simulink model "sm_DynamicCompression"  (R2019b)
settings: Solver=FixedStepDiscrete  StartTime=0.0  StopTime=stop_time  RelTol=1e-3
InitFcn:
  | sm_callback_init
StopFcn:
  | sm_callback_stop
values from neighbouring files (symbols this model uses):
  a = 100*(r^2)    [InitializeCompressionSettings.m]    (also in sm_check_control_signals.m = registers(i).(supplied_fields{j}); sm_check_control_signals_LOCAL_1434.m = registers(i).(supplied_fields{j}))
  B_k_0_init = zeros(1,FIR_0_Uprate)    [sm_callback_init.m]
  B_k_1_init = zeros(1,FIR_0_Uprate)    [sm_callback_init.m]
  B_k_2_init = zeros(1,FIR_0_Uprate)    [sm_callback_init.m]
  B_k_3_init = zeros(1,FIR_0_Uprate)    [sm_callback_init.m]
  B_k_4_init = zeros(1,FIR_0_Uprate)    [sm_callback_init.m]
  B_k_5_init = zeros(1,FIR_0_Uprate)    [sm_callback_init.m]
  calib_bpfs = bpfs    [sm_compression_init.m]
  delayFix = maxDelay-delays    [Initialize_Delay_Values.m]
  F_bits = 28    [TestingLibraryScripts.m]    (also in sm_compression_init.m)
  FIR_0_Size = (ceil(log2(length(calib_bpfs(2:calib_bpfs(1,1)+1 ,1)'))))    [sm_callback_init.m]
  FIR_0_Uprate = 2^FIR_0_Size    [sm_callback_init.m]
  M_bits = 1    [TestingLibraryScripts.m]    (also in sm_compression_init.m = 5)
  M_Bits = M_bits    (= 5)    [sm_compression_init.m]
  mp = sm_init_avalon_signals(mp)    [sm_callback_init.m]
  r_att = nthroot(0.1, s_att)    [sm_compression_init.m]
  r_rel = nthroot(0.1, s_rel)    [sm_compression_init.m]
  recombGain = ones(1,NChans)    [sm_compression_init.m]
  TABLE_SEL_BYPASS_ENABLE = 0    [sm_callback_init.m]
  Ts = mp.Ts    [sm_compression_init.m]
  Ts_system = mp.Ts_system    [sm_compression_init.m]
  W_bits = 32    [TestingLibraryScripts.m]    (also in sm_compression_init.m)
  X_high = 1    [sm_compression_init.m]
undefined symbols (not defined in the file or in its folder): b, c, Gain_Table, ig_eq
libraries: hdlsllib x272, simulink x127, dsphdlfiltering x2
(part 3 of 8)

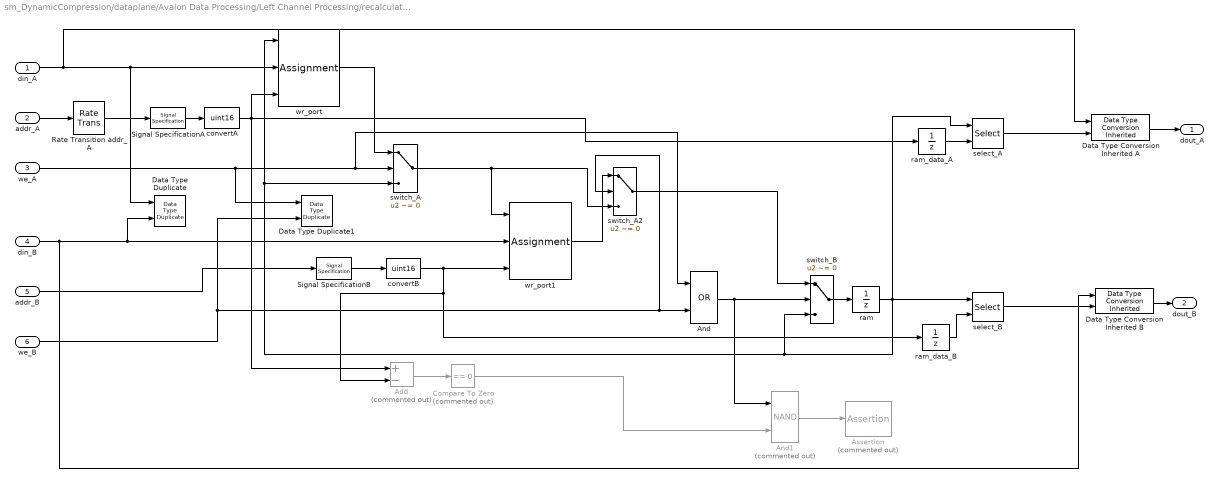
== system sm_DynamicCompression/dataplane/Avalon Data Processing/Left Channel Processing/recalculate/Nchan_FbankAGC_AID/Static_pFIR/Input_Data_Circular_Buffer_old ==
  din_A : Inport
  addr_A : Inport  Port=2
  we_A : Inport  Port=3  OutDataTypeStr=boolean
  din_B : Inport  Port=4
  addr_B : Inport  Port=5
  we_B : Inport  Port=6  OutDataTypeStr=boolean
  Add : Sum  Commented=on  Inputs=+-
  And : Logic  Operator=OR  AllPortsSameDT=off  OutDataTypeStr=boolean
  And1 : Logic  Commented=on  Operator=NAND  AllPortsSameDT=off  OutDataTypeStr=boolean
  Assertion : Assertion  Commented=on  StopWhenAssertionFail=off
  Compare To Zero : simulink/Logic and Bit Operations/Compare To Zero  Commented=on  relop===  OutDataTypeStr=boolean
  Data Type Conversion Inherited A : simulink/Signal Attributes/Data Type Conversion Inherited  ConvertRealWorld=Real World Value  DoSatur=off
      settings: SourceProductName=Simulink  SourceProductBaseCode=SL
  Data Type Conversion Inherited B : simulink/Signal Attributes/Data Type Conversion Inherited  ConvertRealWorld=Real World Value  DoSatur=off
      settings: SourceProductName=Simulink  SourceProductBaseCode=SL
  Data Type Duplicate : DataTypeDuplicate
  Data Type Duplicate1 : DataTypeDuplicate
  Rate Transition addr_A : RateTransition
  Signal SpecificationA : SignalSpecification  OutDataTypeStr=fixdt(0,ram_size,0)  Dimensions=1
  Signal SpecificationB : SignalSpecification  OutDataTypeStr=fixdt(0,ram_size,0)  Dimensions=1
  convertA : DataTypeConversion  OutDataTypeStr=uint16
  convertB : DataTypeConversion  OutDataTypeStr=uint16
  ram : UnitDelay  SampleTime=-1  HasFrameUpgradeWarning=on
  ram_data_A : UnitDelay  SampleTime=-1  HasFrameUpgradeWarning=on
  ram_data_B : UnitDelay  SampleTime=-1  HasFrameUpgradeWarning=on
  select_A : Selector  IndexMode=Zero-based  InputPortWidth=2^ram_size  IndexOptions=Index vector (port)  Indices=[1 3]  OutputSizes=1
  select_B : Selector  IndexMode=Zero-based  InputPortWidth=2^ram_size  IndexOptions=Index vector (port)  Indices=[1 3]  OutputSizes=1
  switch_A : Switch  Criteria=u2 ~= 0
  switch_A2 : Switch  Criteria=u2 ~= 0
  switch_B : Switch  Criteria=u2 ~= 0
  wr_port : Assignment  IndexMode=Zero-based  IndexOptions=Index vector (port)  Indices=1  OutputSizes=[1 1]
  wr_port1 : Assignment  IndexMode=Zero-based  IndexOptions=Index vector (port)  Indices=1  OutputSizes=[1 1]
  dout_A : Outport  VectorParamsAs1DForOutWhenUnconnected=off
  dout_B : Outport  Port=2  VectorParamsAs1DForOutWhenUnconnected=off
  wires:
  Data Type Conversion Inherited A/1 -> dout_A/1
  select_A/1 -> Data Type Conversion Inherited A/2
  Data Type Conversion Inherited B/1 -> dout_B/1
  select_B/1 -> Data Type Conversion Inherited B/2
  Rate Transition addr_A/1 -> Signal SpecificationA/1
  addr_A/1 -> Rate Transition addr_A/1
  din_B/1 -> Data Type Duplicate/2, wr_port1/2, Data Type Conversion Inherited B/1
  convertB/1 -> wr_port1/3, Add/2, ram_data_B/1
  din_A/1 -> wr_port/2, Data Type Duplicate/1, Data Type Conversion Inherited A/1
  ram_data_A/1 -> select_A/2
  we_A/1 -> switch_A/2, And/1, Data Type Duplicate1/1
  ram_data_B/1 -> select_B/2
  addr_B/1 -> Signal SpecificationB/1
  switch_A/1 -> switch_A2/3, wr_port1/1
  we_B/1 -> Data Type Duplicate1/2, And/2, switch_A2/2
  Compare To Zero/1 -> And1/2
  Add/1 -> Compare To Zero/1
  wr_port1/1 -> switch_A2/1
  And/1 -> switch_B/2, And1/1
  wr_port/1 -> switch_A/1
  ram/1 -> select_A/1, wr_port/1, switch_A/3, switch_B/3, select_B/1
  convertA/1 -> Add/1, wr_port/3, ram_data_A/1
  switch_B/1 -> ram/1
  Signal SpecificationB/1 -> convertB/1
  Signal SpecificationA/1 -> convertA/1
  And1/1 -> Assertion/1
  switch_A2/1 -> switch_B/1

== system sm_DynamicCompression/dataplane/Avalon Data Processing/Left Channel Processing/recalculate/Nchan_FbankAGC_AID/Static_pFIR/Multiply_And_Sum ==
  note: Try to use this at some point?
  note: End_of_sample_calc triggers this subsystem to give the FIR output for this sample.
      | Also, it resets the sum memory back to 0.
  x[n-i] : Inport
  End_of_sample_calc : Inport  Port=2
  b_i : Inport  Port=3
  Bitwise Operator : simulink/Logic and Bit Operations/Bitwise Operator  logicop=NOT  UseBitMask=off  BitMask=bin2dec('11011001')  BitMaskRealWorld=Stored Integer
  Constant : Constant  Value=0  OutDataTypeStr=fixdt(1, W_bits, F_bits)  SampleTime=Ts/FIR_0_Uprate
  Multiply-Add : hdlsllib/HDL Operations/Multiply-Add  Function=c+(a.*b)  datatype=Inherit: Same as first input  DoSatur=off  FMA=off
      settings: SourceProductName=Simulink  SourceProductBaseCode=SL
  Reset_Switch : Switch  Criteria=u2 ~= 0  ZeroCross=off
  Sum_memory : UnitDelay  SampleTime=-1  HasFrameUpgradeWarning=on
  Filtered_Output : Outport  VectorParamsAs1DForOutWhenUnconnected=off
  Output_Valid : Outport  Port=2  VectorParamsAs1DForOutWhenUnconnected=off
  wires:
  x[n-i]/1 -> Multiply-Add/1
  End_of_sample_calc/1 -> Output_Valid/1, Bitwise Operator/1
  b_i/1 -> Multiply-Add/2
  Sum_memory/1 -> Multiply-Add/3, Filtered_Output/1
  Multiply-Add/1 -> Reset_Switch/1
  Reset_Switch/1 -> Sum_memory/1
  Constant/1 -> Reset_Switch/3
  Bitwise Operator/1 -> Reset_Switch/2

== system sm_DynamicCompression/dataplane/Avalon Data Processing/Left Channel Processing/recalculate/Nchan_FbankAGC_AID/Static_pFIR1/Addr_Gen  ==
  note: Realign Delay here?
  Add : Sum  OutDataTypeStr=Inherit: Same as first input
  Compare To Zero : simulink/Logic and Bit Operations/Compare To Zero  relop===  OutDataTypeStr=boolean  ZeroCross=off
  Constant : Constant  OutDataTypeStr=fixdt(0, FIR_0_Size,0)  SampleTime=-1
  Counter 0 to |b_k|-1 : simulink/Sources/Counter Free-Running  NumBits=FIR_0_Size  tsamp=Ts/FIR_0_Uprate
  Input_Addr_Counter : simulink/Sources/Counter Free-Running  NumBits=FIR_0_Size  tsamp=Ts
  Rate Transition : RateTransition  OutPortSampleTime=Ts/FIR_0_Uprate
  Realignment_delay : Constant  Value=delayFix(2)  OutDataTypeStr=fixdt(0, FIR_0_Size,0)  SampleTime=-1
  Subtract : Sum  Inputs=+--  OutDataTypeStr=Inherit: Same as first input
  Input_Addr : Outport  VectorParamsAs1DForOutWhenUnconnected=off
  Data_History_Rd_addr : Outport  Port=2  VectorParamsAs1DForOutWhenUnconnected=off
  End_of_sample_calc : Outport  Port=3  VectorParamsAs1DForOutWhenUnconnected=off
  b_k_addr : Outport  Port=4  VectorParamsAs1DForOutWhenUnconnected=off
  wires:
  Rate Transition/1 -> Add/1, Subtract/1
  Compare To Zero/1 -> End_of_sample_calc/1
  Realignment_delay/1 -> Subtract/3
  Constant/1 -> Add/2
  Add/1 -> Input_Addr/1
  Input_Addr_Counter/1 -> Rate Transition/1
  Subtract/1 -> Data_History_Rd_addr/1
  Counter 0 to |b_k|-1/1 -> b_k_addr/1, Compare To Zero/1, Subtract/2

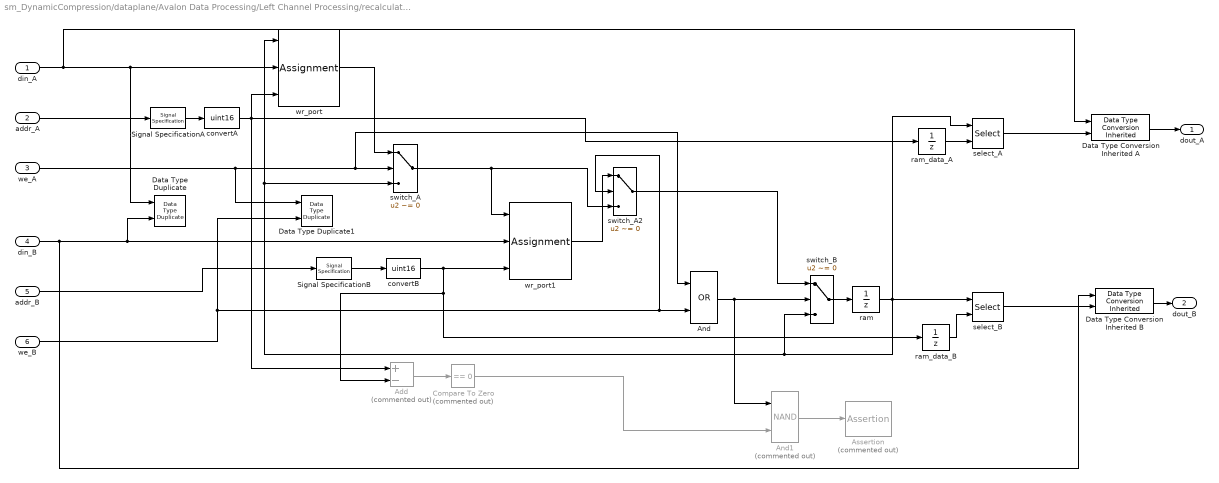
== system sm_DynamicCompression/dataplane/Avalon Data Processing/Left Channel Processing/recalculate/Nchan_FbankAGC_AID/Static_pFIR1/B_k_Memory_Block ==
  din_A : Inport
  addr_A : Inport  Port=2
  we_A : Inport  Port=3  OutDataTypeStr=boolean
  din_B : Inport  Port=4
  addr_B : Inport  Port=5
  we_B : Inport  Port=6  OutDataTypeStr=boolean
  Add : Sum  Commented=on  Inputs=+-
  And : Logic  Operator=OR  AllPortsSameDT=off  OutDataTypeStr=boolean
  And1 : Logic  Commented=on  Operator=NAND  AllPortsSameDT=off  OutDataTypeStr=boolean
  Assertion : Assertion  Commented=on  StopWhenAssertionFail=off
  Compare To Zero : simulink/Logic and Bit Operations/Compare To Zero  Commented=on  relop===  OutDataTypeStr=boolean
  Data Type Conversion Inherited A : simulink/Signal Attributes/Data Type Conversion Inherited  ConvertRealWorld=Real World Value  DoSatur=off
      settings: SourceProductName=Simulink  SourceProductBaseCode=SL
  Data Type Conversion Inherited B : simulink/Signal Attributes/Data Type Conversion Inherited  ConvertRealWorld=Real World Value  DoSatur=off
      settings: SourceProductName=Simulink  SourceProductBaseCode=SL
  Data Type Duplicate : DataTypeDuplicate
  Data Type Duplicate1 : DataTypeDuplicate
  Signal SpecificationA : SignalSpecification  OutDataTypeStr=fixdt(0,ram_size,0)  Dimensions=1
  Signal SpecificationB : SignalSpecification  OutDataTypeStr=fixdt(0,ram_size,0)  Dimensions=1
  convertA : DataTypeConversion  OutDataTypeStr=uint16
  convertB : DataTypeConversion  OutDataTypeStr=uint16
  ram : UnitDelay  InitialCondition=B_k_1_init  SampleTime=-1  HasFrameUpgradeWarning=on
  ram_data_A : UnitDelay  SampleTime=-1  HasFrameUpgradeWarning=on
  ram_data_B : UnitDelay  SampleTime=-1  HasFrameUpgradeWarning=on
  select_A : Selector  IndexMode=Zero-based  InputPortWidth=2^ram_size  IndexOptions=Index vector (port)  Indices=[1 3]  OutputSizes=1
  select_B : Selector  IndexMode=Zero-based  InputPortWidth=2^ram_size  IndexOptions=Index vector (port)  Indices=[1 3]  OutputSizes=1
  switch_A : Switch  Criteria=u2 ~= 0
  switch_A2 : Switch  Criteria=u2 ~= 0
  switch_B : Switch  Criteria=u2 ~= 0
  wr_port : Assignment  IndexMode=Zero-based  IndexOptions=Index vector (port)  Indices=1  OutputSizes=[1 1]
  wr_port1 : Assignment  IndexMode=Zero-based  IndexOptions=Index vector (port)  Indices=1  OutputSizes=[1 1]
  dout_A : Outport  VectorParamsAs1DForOutWhenUnconnected=off
  dout_B : Outport  Port=2  VectorParamsAs1DForOutWhenUnconnected=off
  wires:
  Data Type Conversion Inherited A/1 -> dout_A/1
  select_A/1 -> Data Type Conversion Inherited A/2
  Data Type Conversion Inherited B/1 -> dout_B/1
  select_B/1 -> Data Type Conversion Inherited B/2
  addr_A/1 -> Signal SpecificationA/1
  din_B/1 -> Data Type Conversion Inherited B/1, Data Type Duplicate/2, wr_port1/2
  convertB/1 -> wr_port1/3, Add/2, ram_data_B/1
  din_A/1 -> Data Type Conversion Inherited A/1, wr_port/2, Data Type Duplicate/1
  ram_data_A/1 -> select_A/2
  we_A/1 -> switch_A/2, And/1, Data Type Duplicate1/1
  ram_data_B/1 -> select_B/2
  addr_B/1 -> Signal SpecificationB/1
  switch_A/1 -> switch_A2/3, wr_port1/1
  we_B/1 -> Data Type Duplicate1/2, And/2, switch_A2/2
  Compare To Zero/1 -> And1/2
  Add/1 -> Compare To Zero/1
  wr_port1/1 -> switch_A2/1
  And/1 -> switch_B/2, And1/1
  wr_port/1 -> switch_A/1
  ram/1 -> select_A/1, wr_port/1, switch_A/3, switch_B/3, select_B/1
  convertA/1 -> Add/1, wr_port/3, ram_data_A/1
  switch_B/1 -> ram/1
  Signal SpecificationB/1 -> convertB/1
  Signal SpecificationA/1 -> convertA/1
  And1/1 -> Assertion/1
  switch_A2/1 -> switch_B/1

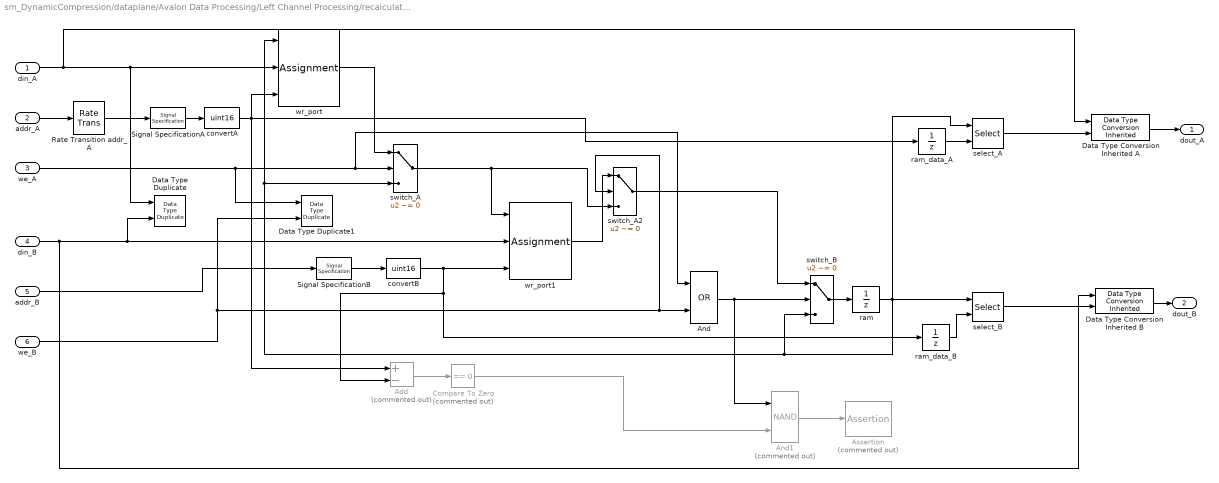
== system sm_DynamicCompression/dataplane/Avalon Data Processing/Left Channel Processing/recalculate/Nchan_FbankAGC_AID/Static_pFIR1/Input_Data_Circular_Buffer_old ==
  din_A : Inport
  addr_A : Inport  Port=2
  we_A : Inport  Port=3  OutDataTypeStr=boolean
  din_B : Inport  Port=4
  addr_B : Inport  Port=5
  we_B : Inport  Port=6  OutDataTypeStr=boolean
  Add : Sum  Commented=on  Inputs=+-
  And : Logic  Operator=OR  AllPortsSameDT=off  OutDataTypeStr=boolean
  And1 : Logic  Commented=on  Operator=NAND  AllPortsSameDT=off  OutDataTypeStr=boolean
  Assertion : Assertion  Commented=on  StopWhenAssertionFail=off
  Compare To Zero : simulink/Logic and Bit Operations/Compare To Zero  Commented=on  relop===  OutDataTypeStr=boolean
  Data Type Conversion Inherited A : simulink/Signal Attributes/Data Type Conversion Inherited  ConvertRealWorld=Real World Value  DoSatur=off
      settings: SourceProductName=Simulink  SourceProductBaseCode=SL
  Data Type Conversion Inherited B : simulink/Signal Attributes/Data Type Conversion Inherited  ConvertRealWorld=Real World Value  DoSatur=off
      settings: SourceProductName=Simulink  SourceProductBaseCode=SL
  Data Type Duplicate : DataTypeDuplicate
  Data Type Duplicate1 : DataTypeDuplicate
  Rate Transition addr_A : RateTransition
  Signal SpecificationA : SignalSpecification  OutDataTypeStr=fixdt(0,ram_size,0)  Dimensions=1
  Signal SpecificationB : SignalSpecification  OutDataTypeStr=fixdt(0,ram_size,0)  Dimensions=1
  convertA : DataTypeConversion  OutDataTypeStr=uint16
  convertB : DataTypeConversion  OutDataTypeStr=uint16
  ram : UnitDelay  SampleTime=-1  HasFrameUpgradeWarning=on
  ram_data_A : UnitDelay  SampleTime=-1  HasFrameUpgradeWarning=on
  ram_data_B : UnitDelay  SampleTime=-1  HasFrameUpgradeWarning=on
  select_A : Selector  IndexMode=Zero-based  InputPortWidth=2^ram_size  IndexOptions=Index vector (port)  Indices=[1 3]  OutputSizes=1
  select_B : Selector  IndexMode=Zero-based  InputPortWidth=2^ram_size  IndexOptions=Index vector (port)  Indices=[1 3]  OutputSizes=1
  switch_A : Switch  Criteria=u2 ~= 0
  switch_A2 : Switch  Criteria=u2 ~= 0
  switch_B : Switch  Criteria=u2 ~= 0
  wr_port : Assignment  IndexMode=Zero-based  IndexOptions=Index vector (port)  Indices=1  OutputSizes=[1 1]
  wr_port1 : Assignment  IndexMode=Zero-based  IndexOptions=Index vector (port)  Indices=1  OutputSizes=[1 1]
  dout_A : Outport  VectorParamsAs1DForOutWhenUnconnected=off
  dout_B : Outport  Port=2  VectorParamsAs1DForOutWhenUnconnected=off
  wires:
  switch_A2/1 -> switch_B/1
  And1/1 -> Assertion/1
  Signal SpecificationA/1 -> convertA/1
  Signal SpecificationB/1 -> convertB/1
  switch_B/1 -> ram/1
  convertA/1 -> ram_data_A/1, wr_port/3, Add/1
  ram/1 -> select_B/1, switch_B/3, switch_A/3, wr_port/1, select_A/1
  wr_port/1 -> switch_A/1
  And/1 -> And1/1, switch_B/2
  wr_port1/1 -> switch_A2/1
  Add/1 -> Compare To Zero/1
  Compare To Zero/1 -> And1/2
  we_B/1 -> switch_A2/2, And/2, Data Type Duplicate1/2
  switch_A/1 -> wr_port1/1, switch_A2/3
  addr_B/1 -> Signal SpecificationB/1
  ram_data_B/1 -> select_B/2
  we_A/1 -> Data Type Duplicate1/1, And/1, switch_A/2
  ram_data_A/1 -> select_A/2
  din_A/1 -> Data Type Conversion Inherited A/1, Data Type Duplicate/1, wr_port/2
  convertB/1 -> ram_data_B/1, Add/2, wr_port1/3
  din_B/1 -> Data Type Conversion Inherited B/1, wr_port1/2, Data Type Duplicate/2
  addr_A/1 -> Rate Transition addr_A/1
  Rate Transition addr_A/1 -> Signal SpecificationA/1
  select_B/1 -> Data Type Conversion Inherited B/2
  Data Type Conversion Inherited B/1 -> dout_B/1
  select_A/1 -> Data Type Conversion Inherited A/2
  Data Type Conversion Inherited A/1 -> dout_A/1

== system sm_DynamicCompression/dataplane/Avalon Data Processing/Left Channel Processing/recalculate/Nchan_FbankAGC_AID/Static_pFIR1/Multiply_And_Sum ==
  note: End_of_sample_calc triggers this subsystem to give the FIR output for this sample.
      | Also, it resets the sum memory back to 0.
  note: Try to use this at some point?
  x[n-i] : Inport
  End_of_sample_calc : Inport  Port=2
  b_i : Inport  Port=3
  Bitwise Operator : simulink/Logic and Bit Operations/Bitwise Operator  logicop=NOT  UseBitMask=off  BitMask=bin2dec('11011001')  BitMaskRealWorld=Stored Integer
  Constant : Constant  Value=0  OutDataTypeStr=fixdt(1, W_bits, F_bits)  SampleTime=Ts/FIR_0_Uprate
  Multiply-Add : hdlsllib/HDL Operations/Multiply-Add  Function=c+(a.*b)  datatype=Inherit: Same as first input  DoSatur=off  FMA=off
      settings: SourceProductName=Simulink  SourceProductBaseCode=SL
  Reset_Switch : Switch  Criteria=u2 ~= 0  ZeroCross=off
  Sum_memory : UnitDelay  SampleTime=-1  HasFrameUpgradeWarning=on
  Filtered_Output : Outport  VectorParamsAs1DForOutWhenUnconnected=off
  Output_Valid : Outport  Port=2  VectorParamsAs1DForOutWhenUnconnected=off
  wires:
  Bitwise Operator/1 -> Reset_Switch/2
  Constant/1 -> Reset_Switch/3
  Reset_Switch/1 -> Sum_memory/1
  Multiply-Add/1 -> Reset_Switch/1
  Sum_memory/1 -> Filtered_Output/1, Multiply-Add/3
  b_i/1 -> Multiply-Add/2
  End_of_sample_calc/1 -> Bitwise Operator/1, Output_Valid/1
  x[n-i]/1 -> Multiply-Add/1

== system sm_DynamicCompression/dataplane/Avalon Data Processing/Left Channel Processing/recalculate/Nchan_FbankAGC_AID/Static_pFIR2/Addr_Gen  ==
  note: Realign Delay here?
  Add : Sum  OutDataTypeStr=Inherit: Same as first input
  Compare To Zero : simulink/Logic and Bit Operations/Compare To Zero  relop===  OutDataTypeStr=boolean  ZeroCross=off
  Constant : Constant  OutDataTypeStr=fixdt(0, FIR_0_Size,0)  SampleTime=-1
  Counter 0 to |b_k|-1 : simulink/Sources/Counter Free-Running  NumBits=FIR_0_Size  tsamp=Ts/FIR_0_Uprate
  Input_Addr_Counter : simulink/Sources/Counter Free-Running  NumBits=FIR_0_Size  tsamp=Ts
  Rate Transition : RateTransition  OutPortSampleTime=Ts/FIR_0_Uprate
  Realignment_delay : Constant  Value=delayFix(3)  OutDataTypeStr=fixdt(0, FIR_0_Size,0)  SampleTime=-1
  Subtract : Sum  Inputs=+--  OutDataTypeStr=Inherit: Same as first input
  Input_Addr : Outport  VectorParamsAs1DForOutWhenUnconnected=off
  Data_History_Rd_addr : Outport  Port=2  VectorParamsAs1DForOutWhenUnconnected=off
  End_of_sample_calc : Outport  Port=3  VectorParamsAs1DForOutWhenUnconnected=off
  b_k_addr : Outport  Port=4  VectorParamsAs1DForOutWhenUnconnected=off
  wires:
  Counter 0 to |b_k|-1/1 -> Subtract/2, Compare To Zero/1, b_k_addr/1
  Subtract/1 -> Data_History_Rd_addr/1
  Input_Addr_Counter/1 -> Rate Transition/1
  Add/1 -> Input_Addr/1
  Constant/1 -> Add/2
  Realignment_delay/1 -> Subtract/3
  Compare To Zero/1 -> End_of_sample_calc/1
  Rate Transition/1 -> Subtract/1, Add/1

== system sm_DynamicCompression/dataplane/Avalon Data Processing/Left Channel Processing/recalculate/Nchan_FbankAGC_AID/Static_pFIR2/B_k_Memory_Block ==
  din_A : Inport
  addr_A : Inport  Port=2
  we_A : Inport  Port=3  OutDataTypeStr=boolean
  din_B : Inport  Port=4
  addr_B : Inport  Port=5
  we_B : Inport  Port=6  OutDataTypeStr=boolean
  Add : Sum  Commented=on  Inputs=+-
  And : Logic  Operator=OR  AllPortsSameDT=off  OutDataTypeStr=boolean
  And1 : Logic  Commented=on  Operator=NAND  AllPortsSameDT=off  OutDataTypeStr=boolean
  Assertion : Assertion  Commented=on  StopWhenAssertionFail=off
  Compare To Zero : simulink/Logic and Bit Operations/Compare To Zero  Commented=on  relop===  OutDataTypeStr=boolean
  Data Type Conversion Inherited A : simulink/Signal Attributes/Data Type Conversion Inherited  ConvertRealWorld=Real World Value  DoSatur=off
      settings: SourceProductName=Simulink  SourceProductBaseCode=SL
  Data Type Conversion Inherited B : simulink/Signal Attributes/Data Type Conversion Inherited  ConvertRealWorld=Real World Value  DoSatur=off
      settings: SourceProductName=Simulink  SourceProductBaseCode=SL
  Data Type Duplicate : DataTypeDuplicate
  Data Type Duplicate1 : DataTypeDuplicate
  Signal SpecificationA : SignalSpecification  OutDataTypeStr=fixdt(0,ram_size,0)  Dimensions=1
  Signal SpecificationB : SignalSpecification  OutDataTypeStr=fixdt(0,ram_size,0)  Dimensions=1
  convertA : DataTypeConversion  OutDataTypeStr=uint16
  convertB : DataTypeConversion  OutDataTypeStr=uint16
  ram : UnitDelay  InitialCondition=B_k_2_init  SampleTime=-1  HasFrameUpgradeWarning=on
  ram_data_A : UnitDelay  SampleTime=-1  HasFrameUpgradeWarning=on
  ram_data_B : UnitDelay  SampleTime=-1  HasFrameUpgradeWarning=on
  select_A : Selector  IndexMode=Zero-based  InputPortWidth=2^ram_size  IndexOptions=Index vector (port)  Indices=[1 3]  OutputSizes=1
  select_B : Selector  IndexMode=Zero-based  InputPortWidth=2^ram_size  IndexOptions=Index vector (port)  Indices=[1 3]  OutputSizes=1
  switch_A : Switch  Criteria=u2 ~= 0
  switch_A2 : Switch  Criteria=u2 ~= 0
  switch_B : Switch  Criteria=u2 ~= 0
  wr_port : Assignment  IndexMode=Zero-based  IndexOptions=Index vector (port)  Indices=1  OutputSizes=[1 1]
  wr_port1 : Assignment  IndexMode=Zero-based  IndexOptions=Index vector (port)  Indices=1  OutputSizes=[1 1]
  dout_A : Outport  VectorParamsAs1DForOutWhenUnconnected=off
  dout_B : Outport  Port=2  VectorParamsAs1DForOutWhenUnconnected=off
  wires:
  switch_A2/1 -> switch_B/1
  And1/1 -> Assertion/1
  Signal SpecificationA/1 -> convertA/1
  Signal SpecificationB/1 -> convertB/1
  switch_B/1 -> ram/1
  convertA/1 -> ram_data_A/1, wr_port/3, Add/1
  ram/1 -> select_B/1, switch_B/3, switch_A/3, wr_port/1, select_A/1
  wr_port/1 -> switch_A/1
  And/1 -> And1/1, switch_B/2
  wr_port1/1 -> switch_A2/1
  Add/1 -> Compare To Zero/1
  Compare To Zero/1 -> And1/2
  we_B/1 -> switch_A2/2, And/2, Data Type Duplicate1/2
  switch_A/1 -> wr_port1/1, switch_A2/3
  addr_B/1 -> Signal SpecificationB/1
  ram_data_B/1 -> select_B/2
  we_A/1 -> Data Type Duplicate1/1, And/1, switch_A/2
  ram_data_A/1 -> select_A/2
  din_A/1 -> Data Type Duplicate/1, wr_port/2, Data Type Conversion Inherited A/1
  convertB/1 -> ram_data_B/1, Add/2, wr_port1/3
  din_B/1 -> wr_port1/2, Data Type Duplicate/2, Data Type Conversion Inherited B/1
  addr_A/1 -> Signal SpecificationA/1
  select_B/1 -> Data Type Conversion Inherited B/2
  Data Type Conversion Inherited B/1 -> dout_B/1
  select_A/1 -> Data Type Conversion Inherited A/2
  Data Type Conversion Inherited A/1 -> dout_A/1

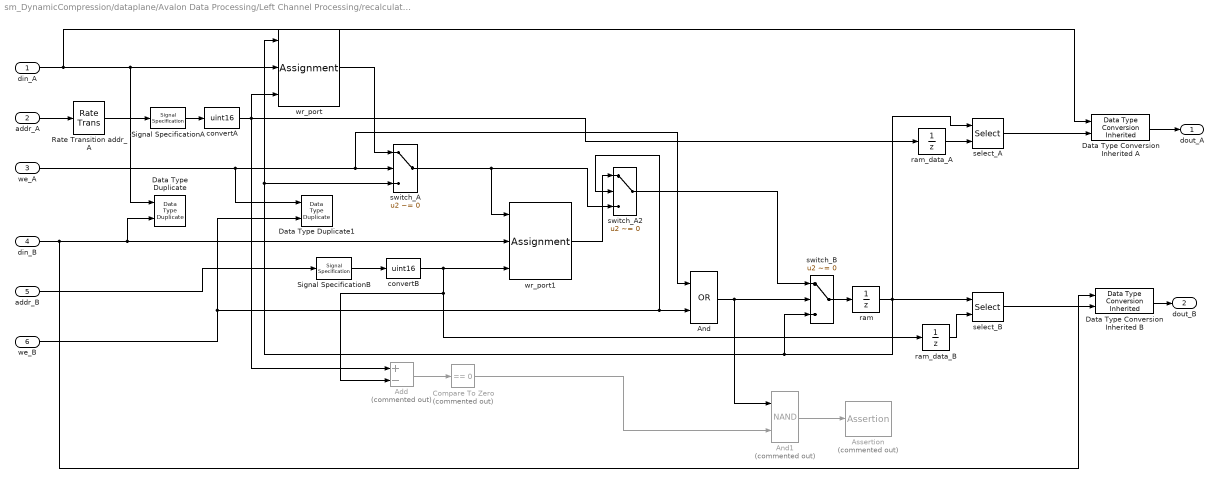
== system sm_DynamicCompression/dataplane/Avalon Data Processing/Left Channel Processing/recalculate/Nchan_FbankAGC_AID/Static_pFIR2/Input_Data_Circular_Buffer_old ==
  din_A : Inport
  addr_A : Inport  Port=2
  we_A : Inport  Port=3  OutDataTypeStr=boolean
  din_B : Inport  Port=4
  addr_B : Inport  Port=5
  we_B : Inport  Port=6  OutDataTypeStr=boolean
  Add : Sum  Commented=on  Inputs=+-
  And : Logic  Operator=OR  AllPortsSameDT=off  OutDataTypeStr=boolean
  And1 : Logic  Commented=on  Operator=NAND  AllPortsSameDT=off  OutDataTypeStr=boolean
  Assertion : Assertion  Commented=on  StopWhenAssertionFail=off
  Compare To Zero : simulink/Logic and Bit Operations/Compare To Zero  Commented=on  relop===  OutDataTypeStr=boolean
  Data Type Conversion Inherited A : simulink/Signal Attributes/Data Type Conversion Inherited  ConvertRealWorld=Real World Value  DoSatur=off
      settings: SourceProductName=Simulink  SourceProductBaseCode=SL
  Data Type Conversion Inherited B : simulink/Signal Attributes/Data Type Conversion Inherited  ConvertRealWorld=Real World Value  DoSatur=off
      settings: SourceProductName=Simulink  SourceProductBaseCode=SL
  Data Type Duplicate : DataTypeDuplicate
  Data Type Duplicate1 : DataTypeDuplicate
  Rate Transition addr_A : RateTransition
  Signal SpecificationA : SignalSpecification  OutDataTypeStr=fixdt(0,ram_size,0)  Dimensions=1
  Signal SpecificationB : SignalSpecification  OutDataTypeStr=fixdt(0,ram_size,0)  Dimensions=1
  convertA : DataTypeConversion  OutDataTypeStr=uint16
  convertB : DataTypeConversion  OutDataTypeStr=uint16
  ram : UnitDelay  SampleTime=-1  HasFrameUpgradeWarning=on
  ram_data_A : UnitDelay  SampleTime=-1  HasFrameUpgradeWarning=on
  ram_data_B : UnitDelay  SampleTime=-1  HasFrameUpgradeWarning=on
  select_A : Selector  IndexMode=Zero-based  InputPortWidth=2^ram_size  IndexOptions=Index vector (port)  Indices=[1 3]  OutputSizes=1
  select_B : Selector  IndexMode=Zero-based  InputPortWidth=2^ram_size  IndexOptions=Index vector (port)  Indices=[1 3]  OutputSizes=1
  switch_A : Switch  Criteria=u2 ~= 0
  switch_A2 : Switch  Criteria=u2 ~= 0
  switch_B : Switch  Criteria=u2 ~= 0
  wr_port : Assignment  IndexMode=Zero-based  IndexOptions=Index vector (port)  Indices=1  OutputSizes=[1 1]
  wr_port1 : Assignment  IndexMode=Zero-based  IndexOptions=Index vector (port)  Indices=1  OutputSizes=[1 1]
  dout_A : Outport  VectorParamsAs1DForOutWhenUnconnected=off
  dout_B : Outport  Port=2  VectorParamsAs1DForOutWhenUnconnected=off
  wires:
  Data Type Conversion Inherited A/1 -> dout_A/1
  select_A/1 -> Data Type Conversion Inherited A/2
  Data Type Conversion Inherited B/1 -> dout_B/1
  select_B/1 -> Data Type Conversion Inherited B/2
  Rate Transition addr_A/1 -> Signal SpecificationA/1
  addr_A/1 -> Rate Transition addr_A/1
  din_B/1 -> Data Type Duplicate/2, wr_port1/2, Data Type Conversion Inherited B/1
  convertB/1 -> wr_port1/3, Add/2, ram_data_B/1
  din_A/1 -> wr_port/2, Data Type Duplicate/1, Data Type Conversion Inherited A/1
  ram_data_A/1 -> select_A/2
  we_A/1 -> switch_A/2, And/1, Data Type Duplicate1/1
  ram_data_B/1 -> select_B/2
  addr_B/1 -> Signal SpecificationB/1
  switch_A/1 -> switch_A2/3, wr_port1/1
  we_B/1 -> Data Type Duplicate1/2, And/2, switch_A2/2
  Compare To Zero/1 -> And1/2
  Add/1 -> Compare To Zero/1
  wr_port1/1 -> switch_A2/1
  And/1 -> switch_B/2, And1/1
  wr_port/1 -> switch_A/1
  ram/1 -> select_A/1, wr_port/1, switch_A/3, switch_B/3, select_B/1
  convertA/1 -> Add/1, wr_port/3, ram_data_A/1
  switch_B/1 -> ram/1
  Signal SpecificationB/1 -> convertB/1
  Signal SpecificationA/1 -> convertA/1
  And1/1 -> Assertion/1
  switch_A2/1 -> switch_B/1

== system sm_DynamicCompression/dataplane/Avalon Data Processing/Left Channel Processing/recalculate/Nchan_FbankAGC_AID/Static_pFIR2/Multiply_And_Sum ==
  note: Try to use this at some point?
  note: End_of_sample_calc triggers this subsystem to give the FIR output for this sample.
      | Also, it resets the sum memory back to 0.
  x[n-i] : Inport
  End_of_sample_calc : Inport  Port=2
  b_i : Inport  Port=3
  Bitwise Operator : simulink/Logic and Bit Operations/Bitwise Operator  logicop=NOT  UseBitMask=off  BitMask=bin2dec('11011001')  BitMaskRealWorld=Stored Integer
  Constant : Constant  Value=0  OutDataTypeStr=fixdt(1, W_bits, F_bits)  SampleTime=Ts/FIR_0_Uprate
  Multiply-Add : hdlsllib/HDL Operations/Multiply-Add  Function=c+(a.*b)  datatype=Inherit: Same as first input  DoSatur=off  FMA=off
      settings: SourceProductName=Simulink  SourceProductBaseCode=SL
  Reset_Switch : Switch  Criteria=u2 ~= 0  ZeroCross=off
  Sum_memory : UnitDelay  SampleTime=-1  HasFrameUpgradeWarning=on
  Filtered_Output : Outport  VectorParamsAs1DForOutWhenUnconnected=off
  Output_Valid : Outport  Port=2  VectorParamsAs1DForOutWhenUnconnected=off
  wires:
  x[n-i]/1 -> Multiply-Add/1
  End_of_sample_calc/1 -> Output_Valid/1, Bitwise Operator/1
  b_i/1 -> Multiply-Add/2
  Sum_memory/1 -> Multiply-Add/3, Filtered_Output/1
  Multiply-Add/1 -> Reset_Switch/1
  Reset_Switch/1 -> Sum_memory/1
  Constant/1 -> Reset_Switch/3
  Bitwise Operator/1 -> Reset_Switch/2

== system sm_DynamicCompression/dataplane/Avalon Data Processing/Left Channel Processing/recalculate/Nchan_FbankAGC_AID/Static_pFIR3/Addr_Gen  ==
  note: Realign Delay here?
  Add : Sum  OutDataTypeStr=Inherit: Same as first input
  Compare To Zero : simulink/Logic and Bit Operations/Compare To Zero  relop===  OutDataTypeStr=boolean  ZeroCross=off
  Constant : Constant  OutDataTypeStr=fixdt(0, FIR_0_Size,0)  SampleTime=-1
  Counter 0 to |b_k|-1 : simulink/Sources/Counter Free-Running  NumBits=FIR_0_Size  tsamp=Ts/FIR_0_Uprate
  Input_Addr_Counter : simulink/Sources/Counter Free-Running  NumBits=FIR_0_Size  tsamp=Ts
  Rate Transition : RateTransition  OutPortSampleTime=Ts/FIR_0_Uprate
  Realignment_delay : Constant  Value=delayFix(4)  OutDataTypeStr=fixdt(0, FIR_0_Size,0)  SampleTime=-1
  Subtract : Sum  Inputs=+--  OutDataTypeStr=Inherit: Same as first input
  Input_Addr : Outport  VectorParamsAs1DForOutWhenUnconnected=off
  Data_History_Rd_addr : Outport  Port=2  VectorParamsAs1DForOutWhenUnconnected=off
  End_of_sample_calc : Outport  Port=3  VectorParamsAs1DForOutWhenUnconnected=off
  b_k_addr : Outport  Port=4  VectorParamsAs1DForOutWhenUnconnected=off
  wires:
  Rate Transition/1 -> Add/1, Subtract/1
  Compare To Zero/1 -> End_of_sample_calc/1
  Realignment_delay/1 -> Subtract/3
  Constant/1 -> Add/2
  Add/1 -> Input_Addr/1
  Input_Addr_Counter/1 -> Rate Transition/1
  Subtract/1 -> Data_History_Rd_addr/1
  Counter 0 to |b_k|-1/1 -> b_k_addr/1, Compare To Zero/1, Subtract/2

== system sm_DynamicCompression/dataplane/Avalon Data Processing/Left Channel Processing/recalculate/Nchan_FbankAGC_AID/Static_pFIR3/B_k_Memory_Block ==
  din_A : Inport
  addr_A : Inport  Port=2
  we_A : Inport  Port=3  OutDataTypeStr=boolean
  din_B : Inport  Port=4
  addr_B : Inport  Port=5
  we_B : Inport  Port=6  OutDataTypeStr=boolean
  Add : Sum  Commented=on  Inputs=+-
  And : Logic  Operator=OR  AllPortsSameDT=off  OutDataTypeStr=boolean
  And1 : Logic  Commented=on  Operator=NAND  AllPortsSameDT=off  OutDataTypeStr=boolean
  Assertion : Assertion  Commented=on  StopWhenAssertionFail=off
  Compare To Zero : simulink/Logic and Bit Operations/Compare To Zero  Commented=on  relop===  OutDataTypeStr=boolean
  Data Type Conversion Inherited A : simulink/Signal Attributes/Data Type Conversion Inherited  ConvertRealWorld=Real World Value  DoSatur=off
      settings: SourceProductName=Simulink  SourceProductBaseCode=SL
  Data Type Conversion Inherited B : simulink/Signal Attributes/Data Type Conversion Inherited  ConvertRealWorld=Real World Value  DoSatur=off
      settings: SourceProductName=Simulink  SourceProductBaseCode=SL
  Data Type Duplicate : DataTypeDuplicate
  Data Type Duplicate1 : DataTypeDuplicate
  Signal SpecificationA : SignalSpecification  OutDataTypeStr=fixdt(0,ram_size,0)  Dimensions=1
  Signal SpecificationB : SignalSpecification  OutDataTypeStr=fixdt(0,ram_size,0)  Dimensions=1
  convertA : DataTypeConversion  OutDataTypeStr=uint16
  convertB : DataTypeConversion  OutDataTypeStr=uint16
  ram : UnitDelay  InitialCondition=B_k_3_init  SampleTime=-1  HasFrameUpgradeWarning=on
  ram_data_A : UnitDelay  SampleTime=-1  HasFrameUpgradeWarning=on
  ram_data_B : UnitDelay  SampleTime=-1  HasFrameUpgradeWarning=on
  select_A : Selector  IndexMode=Zero-based  InputPortWidth=2^ram_size  IndexOptions=Index vector (port)  Indices=[1 3]  OutputSizes=1
  select_B : Selector  IndexMode=Zero-based  InputPortWidth=2^ram_size  IndexOptions=Index vector (port)  Indices=[1 3]  OutputSizes=1
  switch_A : Switch  Criteria=u2 ~= 0
  switch_A2 : Switch  Criteria=u2 ~= 0
  switch_B : Switch  Criteria=u2 ~= 0
  wr_port : Assignment  IndexMode=Zero-based  IndexOptions=Index vector (port)  Indices=1  OutputSizes=[1 1]
  wr_port1 : Assignment  IndexMode=Zero-based  IndexOptions=Index vector (port)  Indices=1  OutputSizes=[1 1]
  dout_A : Outport  VectorParamsAs1DForOutWhenUnconnected=off
  dout_B : Outport  Port=2  VectorParamsAs1DForOutWhenUnconnected=off
  wires:
  Data Type Conversion Inherited A/1 -> dout_A/1
  select_A/1 -> Data Type Conversion Inherited A/2
  Data Type Conversion Inherited B/1 -> dout_B/1
  select_B/1 -> Data Type Conversion Inherited B/2
  addr_A/1 -> Signal SpecificationA/1
  din_B/1 -> Data Type Conversion Inherited B/1, Data Type Duplicate/2, wr_port1/2
  convertB/1 -> wr_port1/3, Add/2, ram_data_B/1
  din_A/1 -> Data Type Conversion Inherited A/1, wr_port/2, Data Type Duplicate/1
  ram_data_A/1 -> select_A/2
  we_A/1 -> switch_A/2, And/1, Data Type Duplicate1/1
  ram_data_B/1 -> select_B/2
  addr_B/1 -> Signal SpecificationB/1
  switch_A/1 -> switch_A2/3, wr_port1/1
  we_B/1 -> Data Type Duplicate1/2, And/2, switch_A2/2
  Compare To Zero/1 -> And1/2
  Add/1 -> Compare To Zero/1
  wr_port1/1 -> switch_A2/1
  And/1 -> switch_B/2, And1/1
  wr_port/1 -> switch_A/1
  ram/1 -> select_A/1, wr_port/1, switch_A/3, switch_B/3, select_B/1
  convertA/1 -> Add/1, wr_port/3, ram_data_A/1
  switch_B/1 -> ram/1
  Signal SpecificationB/1 -> convertB/1
  Signal SpecificationA/1 -> convertA/1
  And1/1 -> Assertion/1
  switch_A2/1 -> switch_B/1

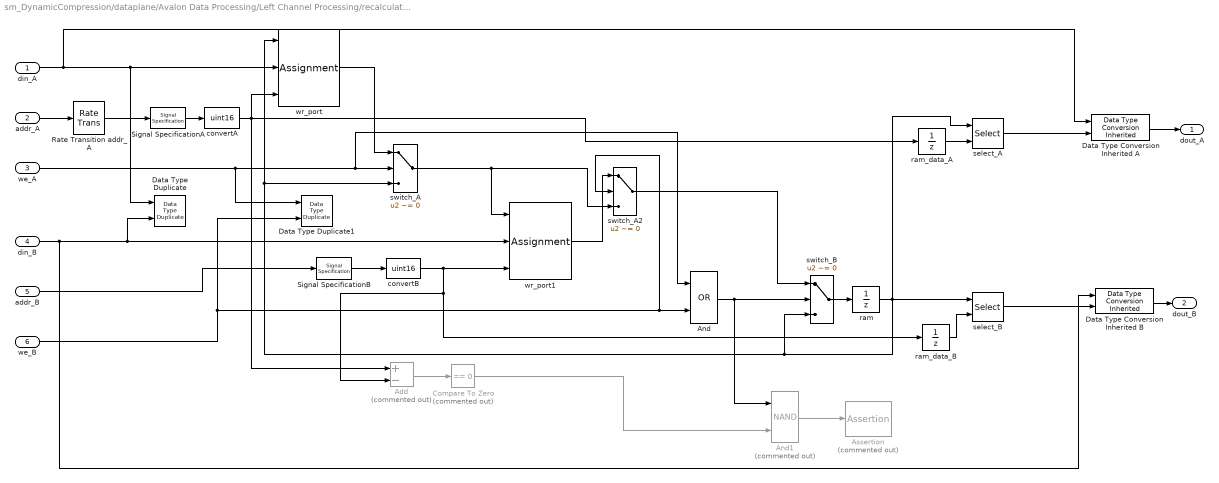
== system sm_DynamicCompression/dataplane/Avalon Data Processing/Left Channel Processing/recalculate/Nchan_FbankAGC_AID/Static_pFIR3/Input_Data_Circular_Buffer_old ==
  din_A : Inport
  addr_A : Inport  Port=2
  we_A : Inport  Port=3  OutDataTypeStr=boolean
  din_B : Inport  Port=4
  addr_B : Inport  Port=5
  we_B : Inport  Port=6  OutDataTypeStr=boolean
  Add : Sum  Commented=on  Inputs=+-
  And : Logic  Operator=OR  AllPortsSameDT=off  OutDataTypeStr=boolean
  And1 : Logic  Commented=on  Operator=NAND  AllPortsSameDT=off  OutDataTypeStr=boolean
  Assertion : Assertion  Commented=on  StopWhenAssertionFail=off
  Compare To Zero : simulink/Logic and Bit Operations/Compare To Zero  Commented=on  relop===  OutDataTypeStr=boolean
  Data Type Conversion Inherited A : simulink/Signal Attributes/Data Type Conversion Inherited  ConvertRealWorld=Real World Value  DoSatur=off
      settings: SourceProductName=Simulink  SourceProductBaseCode=SL
  Data Type Conversion Inherited B : simulink/Signal Attributes/Data Type Conversion Inherited  ConvertRealWorld=Real World Value  DoSatur=off
      settings: SourceProductName=Simulink  SourceProductBaseCode=SL
  Data Type Duplicate : DataTypeDuplicate
  Data Type Duplicate1 : DataTypeDuplicate
  Rate Transition addr_A : RateTransition
  Signal SpecificationA : SignalSpecification  OutDataTypeStr=fixdt(0,ram_size,0)  Dimensions=1
  Signal SpecificationB : SignalSpecification  OutDataTypeStr=fixdt(0,ram_size,0)  Dimensions=1
  convertA : DataTypeConversion  OutDataTypeStr=uint16
  convertB : DataTypeConversion  OutDataTypeStr=uint16
  ram : UnitDelay  SampleTime=-1  HasFrameUpgradeWarning=on
  ram_data_A : UnitDelay  SampleTime=-1  HasFrameUpgradeWarning=on
  ram_data_B : UnitDelay  SampleTime=-1  HasFrameUpgradeWarning=on
  select_A : Selector  IndexMode=Zero-based  InputPortWidth=2^ram_size  IndexOptions=Index vector (port)  Indices=[1 3]  OutputSizes=1
  select_B : Selector  IndexMode=Zero-based  InputPortWidth=2^ram_size  IndexOptions=Index vector (port)  Indices=[1 3]  OutputSizes=1
  switch_A : Switch  Criteria=u2 ~= 0
  switch_A2 : Switch  Criteria=u2 ~= 0
  switch_B : Switch  Criteria=u2 ~= 0
  wr_port : Assignment  IndexMode=Zero-based  IndexOptions=Index vector (port)  Indices=1  OutputSizes=[1 1]
  wr_port1 : Assignment  IndexMode=Zero-based  IndexOptions=Index vector (port)  Indices=1  OutputSizes=[1 1]
  dout_A : Outport  VectorParamsAs1DForOutWhenUnconnected=off
  dout_B : Outport  Port=2  VectorParamsAs1DForOutWhenUnconnected=off
  wires:
  switch_A2/1 -> switch_B/1
  And1/1 -> Assertion/1
  Signal SpecificationA/1 -> convertA/1
  Signal SpecificationB/1 -> convertB/1
  switch_B/1 -> ram/1
  convertA/1 -> ram_data_A/1, wr_port/3, Add/1
  ram/1 -> select_B/1, switch_B/3, switch_A/3, wr_port/1, select_A/1
  wr_port/1 -> switch_A/1
  And/1 -> And1/1, switch_B/2
  wr_port1/1 -> switch_A2/1
  Add/1 -> Compare To Zero/1
  Compare To Zero/1 -> And1/2
  we_B/1 -> switch_A2/2, And/2, Data Type Duplicate1/2
  switch_A/1 -> wr_port1/1, switch_A2/3
  addr_B/1 -> Signal SpecificationB/1
  ram_data_B/1 -> select_B/2
  we_A/1 -> Data Type Duplicate1/1, And/1, switch_A/2
  ram_data_A/1 -> select_A/2
  din_A/1 -> Data Type Conversion Inherited A/1, Data Type Duplicate/1, wr_port/2
  convertB/1 -> ram_data_B/1, Add/2, wr_port1/3
  din_B/1 -> Data Type Conversion Inherited B/1, wr_port1/2, Data Type Duplicate/2
  addr_A/1 -> Rate Transition addr_A/1
  Rate Transition addr_A/1 -> Signal SpecificationA/1
  select_B/1 -> Data Type Conversion Inherited B/2
  Data Type Conversion Inherited B/1 -> dout_B/1
  select_A/1 -> Data Type Conversion Inherited A/2
  Data Type Conversion Inherited A/1 -> dout_A/1

== system sm_DynamicCompression/dataplane/Avalon Data Processing/Left Channel Processing/recalculate/Nchan_FbankAGC_AID/Static_pFIR3/Multiply_And_Sum ==
  note: End_of_sample_calc triggers this subsystem to give the FIR output for this sample.
      | Also, it resets the sum memory back to 0.
  note: Try to use this at some point?
  x[n-i] : Inport
  End_of_sample_calc : Inport  Port=2
  b_i : Inport  Port=3
  Bitwise Operator : simulink/Logic and Bit Operations/Bitwise Operator  logicop=NOT  UseBitMask=off  BitMask=bin2dec('11011001')  BitMaskRealWorld=Stored Integer
  Constant : Constant  Value=0  OutDataTypeStr=fixdt(1, W_bits, F_bits)  SampleTime=Ts/FIR_0_Uprate
  Multiply-Add : hdlsllib/HDL Operations/Multiply-Add  Function=c+(a.*b)  datatype=Inherit: Same as first input  DoSatur=off  FMA=off
      settings: SourceProductName=Simulink  SourceProductBaseCode=SL
  Reset_Switch : Switch  Criteria=u2 ~= 0  ZeroCross=off
  Sum_memory : UnitDelay  SampleTime=-1  HasFrameUpgradeWarning=on
  Filtered_Output : Outport  VectorParamsAs1DForOutWhenUnconnected=off
  Output_Valid : Outport  Port=2  VectorParamsAs1DForOutWhenUnconnected=off
  wires:
  Bitwise Operator/1 -> Reset_Switch/2
  Constant/1 -> Reset_Switch/3
  Reset_Switch/1 -> Sum_memory/1
  Multiply-Add/1 -> Reset_Switch/1
  Sum_memory/1 -> Filtered_Output/1, Multiply-Add/3
  b_i/1 -> Multiply-Add/2
  End_of_sample_calc/1 -> Bitwise Operator/1, Output_Valid/1
  x[n-i]/1 -> Multiply-Add/1

== system sm_DynamicCompression/dataplane/Avalon Data Processing/Left Channel Processing/recalculate/Nchan_FbankAGC_AID/Static_pFIR4/Addr_Gen  ==
  note: Realign Delay here?
  Add : Sum  OutDataTypeStr=Inherit: Same as first input
  Compare To Zero : simulink/Logic and Bit Operations/Compare To Zero  relop===  OutDataTypeStr=boolean  ZeroCross=off
  Constant : Constant  OutDataTypeStr=fixdt(0, FIR_0_Size,0)  SampleTime=-1
  Counter 0 to |b_k|-1 : simulink/Sources/Counter Free-Running  NumBits=FIR_0_Size  tsamp=Ts/FIR_0_Uprate
  Input_Addr_Counter : simulink/Sources/Counter Free-Running  NumBits=FIR_0_Size  tsamp=Ts
  Rate Transition : RateTransition  OutPortSampleTime=Ts/FIR_0_Uprate
  Realignment_delay : Constant  Value=delayFix(5)  OutDataTypeStr=fixdt(0, FIR_0_Size,0)  SampleTime=-1
  Subtract : Sum  Inputs=+--  OutDataTypeStr=Inherit: Same as first input
  Input_Addr : Outport  VectorParamsAs1DForOutWhenUnconnected=off
  Data_History_Rd_addr : Outport  Port=2  VectorParamsAs1DForOutWhenUnconnected=off
  End_of_sample_calc : Outport  Port=3  VectorParamsAs1DForOutWhenUnconnected=off
  b_k_addr : Outport  Port=4  VectorParamsAs1DForOutWhenUnconnected=off
  wires:
  Counter 0 to |b_k|-1/1 -> Subtract/2, Compare To Zero/1, b_k_addr/1
  Subtract/1 -> Data_History_Rd_addr/1
  Input_Addr_Counter/1 -> Rate Transition/1
  Add/1 -> Input_Addr/1
  Constant/1 -> Add/2
  Realignment_delay/1 -> Subtract/3
  Compare To Zero/1 -> End_of_sample_calc/1
  Rate Transition/1 -> Subtract/1, Add/1

== system sm_DynamicCompression/dataplane/Avalon Data Processing/Left Channel Processing/recalculate/Nchan_FbankAGC_AID/Static_pFIR4/B_k_Memory_Block ==
  din_A : Inport
  addr_A : Inport  Port=2
  we_A : Inport  Port=3  OutDataTypeStr=boolean
  din_B : Inport  Port=4
  addr_B : Inport  Port=5
  we_B : Inport  Port=6  OutDataTypeStr=boolean
  Add : Sum  Commented=on  Inputs=+-
  And : Logic  Operator=OR  AllPortsSameDT=off  OutDataTypeStr=boolean
  And1 : Logic  Commented=on  Operator=NAND  AllPortsSameDT=off  OutDataTypeStr=boolean
  Assertion : Assertion  Commented=on  StopWhenAssertionFail=off
  Compare To Zero : simulink/Logic and Bit Operations/Compare To Zero  Commented=on  relop===  OutDataTypeStr=boolean
  Data Type Conversion Inherited A : simulink/Signal Attributes/Data Type Conversion Inherited  ConvertRealWorld=Real World Value  DoSatur=off
      settings: SourceProductName=Simulink  SourceProductBaseCode=SL
  Data Type Conversion Inherited B : simulink/Signal Attributes/Data Type Conversion Inherited  ConvertRealWorld=Real World Value  DoSatur=off
      settings: SourceProductName=Simulink  SourceProductBaseCode=SL
  Data Type Duplicate : DataTypeDuplicate
  Data Type Duplicate1 : DataTypeDuplicate
  Signal SpecificationA : SignalSpecification  OutDataTypeStr=fixdt(0,ram_size,0)  Dimensions=1
  Signal SpecificationB : SignalSpecification  OutDataTypeStr=fixdt(0,ram_size,0)  Dimensions=1
  convertA : DataTypeConversion  OutDataTypeStr=uint16
  convertB : DataTypeConversion  OutDataTypeStr=uint16
  ram : UnitDelay  InitialCondition=B_k_4_init  SampleTime=-1  HasFrameUpgradeWarning=on
  ram_data_A : UnitDelay  SampleTime=-1  HasFrameUpgradeWarning=on
  ram_data_B : UnitDelay  SampleTime=-1  HasFrameUpgradeWarning=on
  select_A : Selector  IndexMode=Zero-based  InputPortWidth=2^ram_size  IndexOptions=Index vector (port)  Indices=[1 3]  OutputSizes=1
  select_B : Selector  IndexMode=Zero-based  InputPortWidth=2^ram_size  IndexOptions=Index vector (port)  Indices=[1 3]  OutputSizes=1
  switch_A : Switch  Criteria=u2 ~= 0
  switch_A2 : Switch  Criteria=u2 ~= 0
  switch_B : Switch  Criteria=u2 ~= 0
  wr_port : Assignment  IndexMode=Zero-based  IndexOptions=Index vector (port)  Indices=1  OutputSizes=[1 1]
  wr_port1 : Assignment  IndexMode=Zero-based  IndexOptions=Index vector (port)  Indices=1  OutputSizes=[1 1]
  dout_A : Outport  VectorParamsAs1DForOutWhenUnconnected=off
  dout_B : Outport  Port=2  VectorParamsAs1DForOutWhenUnconnected=off
  wires:
  switch_A2/1 -> switch_B/1
  And1/1 -> Assertion/1
  Signal SpecificationA/1 -> convertA/1
  Signal SpecificationB/1 -> convertB/1
  switch_B/1 -> ram/1
  convertA/1 -> ram_data_A/1, wr_port/3, Add/1
  ram/1 -> select_B/1, switch_B/3, switch_A/3, wr_port/1, select_A/1
  wr_port/1 -> switch_A/1
  And/1 -> And1/1, switch_B/2
  wr_port1/1 -> switch_A2/1
  Add/1 -> Compare To Zero/1
  Compare To Zero/1 -> And1/2
  we_B/1 -> switch_A2/2, And/2, Data Type Duplicate1/2
  switch_A/1 -> wr_port1/1, switch_A2/3
  addr_B/1 -> Signal SpecificationB/1
  ram_data_B/1 -> select_B/2
  we_A/1 -> Data Type Duplicate1/1, And/1, switch_A/2
  ram_data_A/1 -> select_A/2
  din_A/1 -> Data Type Duplicate/1, wr_port/2, Data Type Conversion Inherited A/1
  convertB/1 -> ram_data_B/1, Add/2, wr_port1/3
  din_B/1 -> wr_port1/2, Data Type Duplicate/2, Data Type Conversion Inherited B/1
  addr_A/1 -> Signal SpecificationA/1
  select_B/1 -> Data Type Conversion Inherited B/2
  Data Type Conversion Inherited B/1 -> dout_B/1
  select_A/1 -> Data Type Conversion Inherited A/2
  Data Type Conversion Inherited A/1 -> dout_A/1

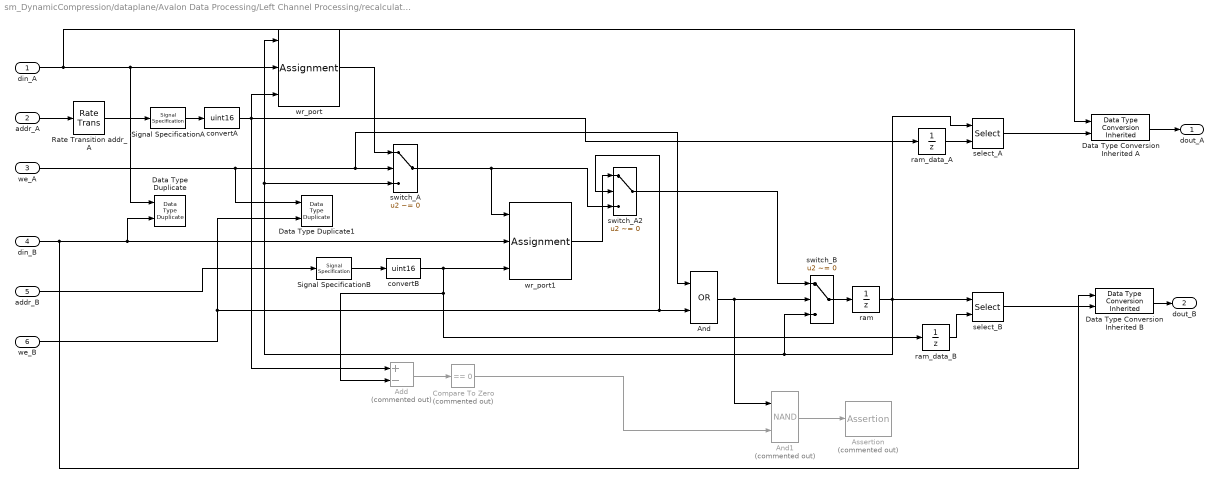
== system sm_DynamicCompression/dataplane/Avalon Data Processing/Left Channel Processing/recalculate/Nchan_FbankAGC_AID/Static_pFIR4/Input_Data_Circular_Buffer_old ==
  din_A : Inport
  addr_A : Inport  Port=2
  we_A : Inport  Port=3  OutDataTypeStr=boolean
  din_B : Inport  Port=4
  addr_B : Inport  Port=5
  we_B : Inport  Port=6  OutDataTypeStr=boolean
  Add : Sum  Commented=on  Inputs=+-
  And : Logic  Operator=OR  AllPortsSameDT=off  OutDataTypeStr=boolean
  And1 : Logic  Commented=on  Operator=NAND  AllPortsSameDT=off  OutDataTypeStr=boolean
  Assertion : Assertion  Commented=on  StopWhenAssertionFail=off
  Compare To Zero : simulink/Logic and Bit Operations/Compare To Zero  Commented=on  relop===  OutDataTypeStr=boolean
  Data Type Conversion Inherited A : simulink/Signal Attributes/Data Type Conversion Inherited  ConvertRealWorld=Real World Value  DoSatur=off
      settings: SourceProductName=Simulink  SourceProductBaseCode=SL
  Data Type Conversion Inherited B : simulink/Signal Attributes/Data Type Conversion Inherited  ConvertRealWorld=Real World Value  DoSatur=off
      settings: SourceProductName=Simulink  SourceProductBaseCode=SL
  Data Type Duplicate : DataTypeDuplicate
  Data Type Duplicate1 : DataTypeDuplicate
  Rate Transition addr_A : RateTransition
  Signal SpecificationA : SignalSpecification  OutDataTypeStr=fixdt(0,ram_size,0)  Dimensions=1
  Signal SpecificationB : SignalSpecification  OutDataTypeStr=fixdt(0,ram_size,0)  Dimensions=1
  convertA : DataTypeConversion  OutDataTypeStr=uint16
  convertB : DataTypeConversion  OutDataTypeStr=uint16
  ram : UnitDelay  SampleTime=-1  HasFrameUpgradeWarning=on
  ram_data_A : UnitDelay  SampleTime=-1  HasFrameUpgradeWarning=on
  ram_data_B : UnitDelay  SampleTime=-1  HasFrameUpgradeWarning=on
  select_A : Selector  IndexMode=Zero-based  InputPortWidth=2^ram_size  IndexOptions=Index vector (port)  Indices=[1 3]  OutputSizes=1
  select_B : Selector  IndexMode=Zero-based  InputPortWidth=2^ram_size  IndexOptions=Index vector (port)  Indices=[1 3]  OutputSizes=1
  switch_A : Switch  Criteria=u2 ~= 0
  switch_A2 : Switch  Criteria=u2 ~= 0
  switch_B : Switch  Criteria=u2 ~= 0
  wr_port : Assignment  IndexMode=Zero-based  IndexOptions=Index vector (port)  Indices=1  OutputSizes=[1 1]
  wr_port1 : Assignment  IndexMode=Zero-based  IndexOptions=Index vector (port)  Indices=1  OutputSizes=[1 1]
  dout_A : Outport  VectorParamsAs1DForOutWhenUnconnected=off
  dout_B : Outport  Port=2  VectorParamsAs1DForOutWhenUnconnected=off
  wires:
  Data Type Conversion Inherited A/1 -> dout_A/1
  select_A/1 -> Data Type Conversion Inherited A/2
  Data Type Conversion Inherited B/1 -> dout_B/1
  select_B/1 -> Data Type Conversion Inherited B/2
  Rate Transition addr_A/1 -> Signal SpecificationA/1
  addr_A/1 -> Rate Transition addr_A/1
  din_B/1 -> Data Type Duplicate/2, wr_port1/2, Data Type Conversion Inherited B/1
  convertB/1 -> wr_port1/3, Add/2, ram_data_B/1
  din_A/1 -> wr_port/2, Data Type Duplicate/1, Data Type Conversion Inherited A/1
  ram_data_A/1 -> select_A/2
  we_A/1 -> switch_A/2, And/1, Data Type Duplicate1/1
  ram_data_B/1 -> select_B/2
  addr_B/1 -> Signal SpecificationB/1
  switch_A/1 -> switch_A2/3, wr_port1/1
  we_B/1 -> Data Type Duplicate1/2, And/2, switch_A2/2
  Compare To Zero/1 -> And1/2
  Add/1 -> Compare To Zero/1
  wr_port1/1 -> switch_A2/1
  And/1 -> switch_B/2, And1/1
  wr_port/1 -> switch_A/1
  ram/1 -> select_A/1, wr_port/1, switch_A/3, switch_B/3, select_B/1
  convertA/1 -> Add/1, wr_port/3, ram_data_A/1
  switch_B/1 -> ram/1
  Signal SpecificationB/1 -> convertB/1
  Signal SpecificationA/1 -> convertA/1
  And1/1 -> Assertion/1
  switch_A2/1 -> switch_B/1

== system sm_DynamicCompression/dataplane/Avalon Data Processing/Left Channel Processing/recalculate/Nchan_FbankAGC_AID/Static_pFIR4/Multiply_And_Sum ==
  note: Try to use this at some point?
  note: End_of_sample_calc triggers this subsystem to give the FIR output for this sample.
      | Also, it resets the sum memory back to 0.
  x[n-i] : Inport
  End_of_sample_calc : Inport  Port=2
  b_i : Inport  Port=3
  Bitwise Operator : simulink/Logic and Bit Operations/Bitwise Operator  logicop=NOT  UseBitMask=off  BitMask=bin2dec('11011001')  BitMaskRealWorld=Stored Integer
  Constant : Constant  Value=0  OutDataTypeStr=fixdt(1, W_bits, F_bits)  SampleTime=Ts/FIR_0_Uprate
  Multiply-Add : hdlsllib/HDL Operations/Multiply-Add  Function=c+(a.*b)  datatype=Inherit: Same as first input  DoSatur=off  FMA=off
      settings: SourceProductName=Simulink  SourceProductBaseCode=SL
  Reset_Switch : Switch  Criteria=u2 ~= 0  ZeroCross=off
  Sum_memory : UnitDelay  SampleTime=-1  HasFrameUpgradeWarning=on
  Filtered_Output : Outport  VectorParamsAs1DForOutWhenUnconnected=off
  Output_Valid : Outport  Port=2  VectorParamsAs1DForOutWhenUnconnected=off
  wires:
  x[n-i]/1 -> Multiply-Add/1
  End_of_sample_calc/1 -> Output_Valid/1, Bitwise Operator/1
  b_i/1 -> Multiply-Add/2
  Sum_memory/1 -> Multiply-Add/3, Filtered_Output/1
  Multiply-Add/1 -> Reset_Switch/1
  Reset_Switch/1 -> Sum_memory/1
  Constant/1 -> Reset_Switch/3
  Bitwise Operator/1 -> Reset_Switch/2

== system sm_DynamicCompression/dataplane/Avalon Data Processing/Left Channel Processing/recalculate/Nchan_FbankAGC_AID/Compression_1/Compression_Envelope/Attack_Envelope ==
  note: ATTACK
  Curr : Inport
  Desired : Inport  Port=2
  Enable : EnablePort
  Product : Product  OutDataTypeStr=Inherit: Same as first input
  Subtract : Sum  Inputs=+-
  Subtract1 : Sum  OutDataTypeStr=fixdt(1,W_bits, F_bits)
  r_att(1) : Constant  Value=r_att(1)  OutDataTypeStr=fixdt(1,W_bits*2,W_bits+F_bits)  SampleTime=-1
  Gain_out : Outport  InitialOutput=0  VectorParamsAs1DForOutWhenUnconnected=off
  wires:
  Desired/1 -> Subtract/2, Subtract1/2
  Curr/1 -> Subtract/1
  Subtract/1 -> Product/2
  r_att(1)/1 -> Product/1
  Product/1 -> Subtract1/1  "Apply_Envelope"
  Subtract1/1 -> Gain_out/1

== system sm_DynamicCompression/dataplane/Avalon Data Processing/Left Channel Processing/recalculate/Nchan_FbankAGC_AID/Compression_1/Compression_Envelope/Release_Envelope ==
  note: RELEASE
  Curr : Inport
  Desired : Inport  Port=2
  Enable : EnablePort
  Product : Product  OutDataTypeStr=Inherit: Same as first input
  Subtract : Sum  Inputs=+-
  Subtract1 : Sum  Inputs=+-  OutDataTypeStr=Inherit: Same as first input
  r_rel(1) : Constant  Value=r_rel(1)  OutDataTypeStr=fixdt(1,W_bits*2,W_bits+F_bits)  SampleTime=-1
  Gain_out : Outport  InitialOutput=0  VectorParamsAs1DForOutWhenUnconnected=off
  wires:
  Desired/1 -> Subtract1/1, Subtract/1
  Curr/1 -> Subtract/2
  Subtract/1 -> Product/1
  r_rel(1)/1 -> Product/2
  Product/1 -> Subtract1/2  "Apply_Envelope"
  Subtract1/1 -> Gain_out/1
